simulink model "TopCsc"  (Simulink 6.3)
settings: Solver=ode45  StartTime=0.0  StopTime=10.0  RelTol=1e-3
InitFcn:
  | %% DSPBuilder Start
  | alt_dspbuilder_update_model(bdroot)
  | %% DSPBuilder End
libraries: allblocks_alteradspbuilder2 x14
settings Model: LastModifiedBy=LKONG  StrictBusMsg=None
settings DataIOCC: SignalLoggingName=sigsOut
settings OptimizationCC: InlineInvariantSignals=on
settings DebuggingCC: SolverPrmCheckMsg=none
settings HardwareCC: TargetUnknown=on

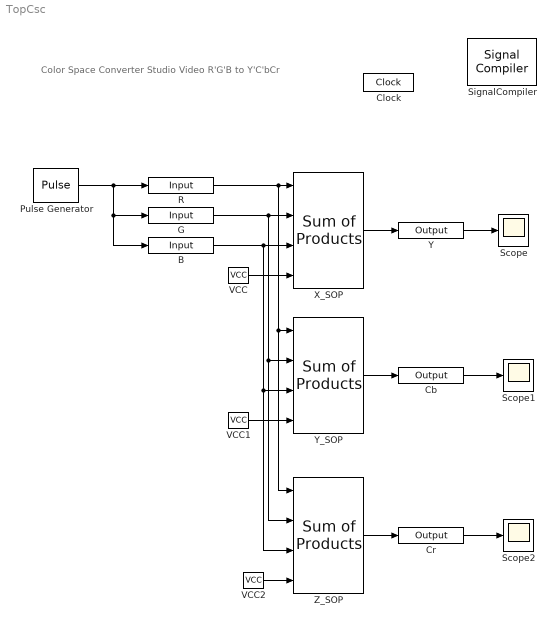
== system TopCsc ==
  note: Color Space Converter
      | Studio Video R'G'B to Y'C'bCr
  B : allblocks_alteradspbuilder2/Input  iofile=D:\dspbuilder\dspb_71\DesignExamples\demos\Transforms\Csc\tb_TopCsc\TopCsc_B.salt  BusType=Signed Integer  bwl=8  bwr=0  SpecifyClock=off  PORTTYPE=Input
  Cb : allblocks_alteradspbuilder2/Output  iofile=D:\dspbuilder\dspb_71\DesignExamples\demos\Transforms\Csc\tb_TopCsc\TopCsc_Cb.capture  BusType=Signed Integer  bwl=26  bwr=0  PORTTYPE=Output
  Clock : allblocks_alteradspbuilder2/Clock  ClockPeriod=100  ClockPeriodUnit=ns  SampleTime=1  SimulationStartCycle=5  PhaseOffset=0  Reset=aclr  Export=off
  Cr : allblocks_alteradspbuilder2/Output  iofile=D:\dspbuilder\dspb_71\DesignExamples\demos\Transforms\Csc\tb_TopCsc\TopCsc_Cr.capture  BusType=Signed Integer  bwl=26  bwr=0  PORTTYPE=Output
  G : allblocks_alteradspbuilder2/Input  iofile=D:\dspbuilder\dspb_71\DesignExamples\demos\Transforms\Csc\tb_TopCsc\TopCsc_G.salt  BusType=Signed Integer  bwl=8  bwr=0  SpecifyClock=off  PORTTYPE=Input
  Pulse Generator : DiscretePulseGenerator  Amplitude=120  Period=200
  R : allblocks_alteradspbuilder2/Input  iofile=D:\dspbuilder\dspb_71\DesignExamples\demos\Transforms\Csc\tb_TopCsc\TopCsc_R.salt  BusType=Signed Integer  bwl=8  bwr=0  SpecifyClock=off  PORTTYPE=Input
  Scope : Scope
  Scope1 : Scope
  Scope2 : Scope
      settings: SaveName=ScopeData2
  SignalCompiler : allblocks_alteradspbuilder2/Signal Compiler  DeviceFamily=Stratix IV  DeviceName=AUTO  EnableSignalTap=off  SignalTapDepth=128  UseBoardBlock=off  StpUseDefaultClock=on  StpClock=Clock
  VCC : allblocks_alteradspbuilder2/VCC  SpecifyClock=off
  VCC1 : allblocks_alteradspbuilder2/VCC  SpecifyClock=off
  VCC2 : allblocks_alteradspbuilder2/VCC  SpecifyClock=off
  X_SOP : allblocks_alteradspbuilder2/Sum of Products  BusType=Signed Integer  InputBwl=8  InputBwr=0  number_of_coefficients=4  CoefBwl=16  CoefBwr=0  coefficients=[39 75 14 2048]  pipeline=4  full_resolution=on  OutputBwl=(26) - (0)  OutputBwr=0  TruncateLsb=0  implementation=Auto  use_ena=off  use_aclr=off
  Y : allblocks_alteradspbuilder2/Output  iofile=D:\dspbuilder\dspb_71\DesignExamples\demos\Transforms\Csc\tb_TopCsc\TopCsc_Y.capture  BusType=Signed Integer  bwl=26  bwr=0  PORTTYPE=Output
  Y_SOP : allblocks_alteradspbuilder2/Sum of Products  BusType=Signed Integer  InputBwl=8  InputBwr=0  number_of_coefficients=4  CoefBwl=16  CoefBwr=0  coefficients=[-22 -44 66 16384]  pipeline=4  full_resolution=on  OutputBwl=(26) - (0)  OutputBwr=0  TruncateLsb=0  implementation=Auto  use_ena=off  use_aclr=off
  Z_SOP : allblocks_alteradspbuilder2/Sum of Products  BusType=Signed Integer  InputBwl=8  InputBwr=0  number_of_coefficients=4  CoefBwl=16  CoefBwr=0  coefficients=[66 -55 -10 16384]  pipeline=4  full_resolution=on  OutputBwl=(26) - (0)  OutputBwr=0  TruncateLsb=0  implementation=Auto  use_ena=off  use_aclr=off
  wires:
  R/1 -> X_SOP/1, Y_SOP/1, Z_SOP/1
  G/1 -> X_SOP/2, Y_SOP/2, Z_SOP/2
  B/1 -> X_SOP/3, Y_SOP/3, Z_SOP/3
  VCC/1 -> X_SOP/4
  VCC1/1 -> Y_SOP/4
  VCC2/1 -> Z_SOP/4
  X_SOP/1 -> Y/1
  Y_SOP/1 -> Cb/1
  Z_SOP/1 -> Cr/1
  Pulse Generator/1 -> R/1, G/1, B/1
  Y/1 -> Scope/1
  Cb/1 -> Scope1/1
  Cr/1 -> Scope2/1
